simulink model "Rozmyty"  (R2017b)
settings: Solver=ode1  StartTime=0.0  StopTime=3  FixedStep=0.0001  RelTol=1e-3
values from neighbouring files (symbols this model uses):
  Te = 0.001    [Dane_rozmyte.m]
  Tm = 0.2    [Dane_rozmyte.m]
libraries: fuzblock x48
settings Model: Creator=kamil  LastModifiedBy=kamil

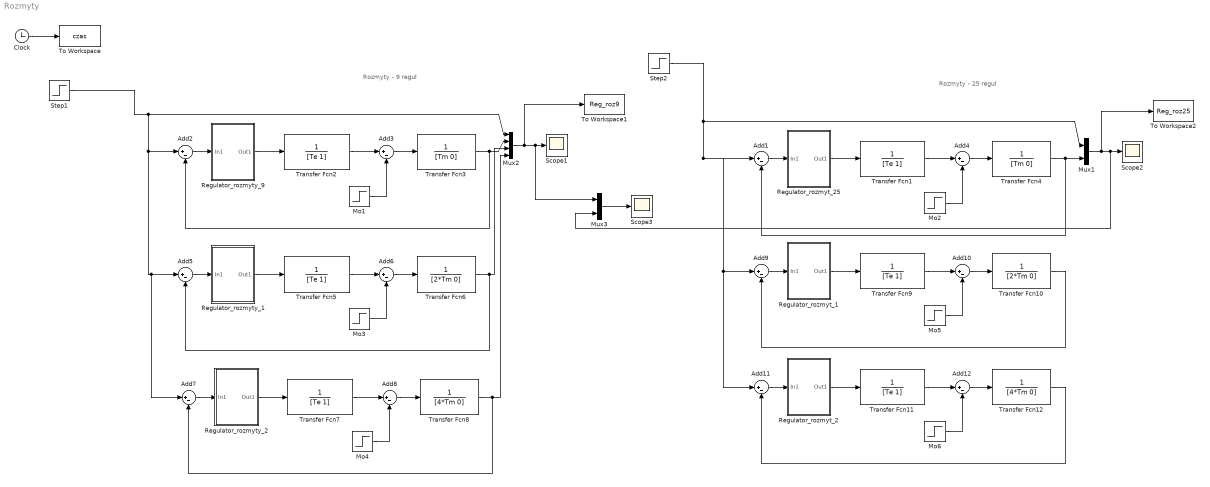
== system Rozmyty ==
  note: Rozmyty - 9 reguł
  note: Rozmyty - 25 reguł
  Add{1..12} (12 alike) : Sum  Inputs=|+-
  Clock : Clock
  Mo{1..6} (6 alike) : Step  Time=2  After=0.5  SampleTime=0
  Mux1 : Mux  Inputs=2
  Mux2 : Mux
  Mux3 : Mux  Inputs=2
  Regulator_rozmyt_1 : Subsystem
  Regulator_rozmyt_2 : Subsystem
  Regulator_rozmyt_25 : Subsystem
  Regulator_rozmyty_1 : Subsystem
  Regulator_rozmyty_2 : Subsystem
  Regulator_rozmyty_9 : Subsystem
  Scope1 : Scope
  Scope2 : Scope
  Scope3 : Scope
  Step1 : Step  After=0.25  SampleTime=0
  Step2 : Step  After=0.25  SampleTime=0
  To Workspace : ToWorkspace  VariableName=czas  SampleTime=-1
  To Workspace1 : ToWorkspace  VariableName=Reg_roz9  SampleTime=-1
  To Workspace2 : ToWorkspace  VariableName=Reg_roz25  SampleTime=-1
  Transfer Fcn{1..2,5,7,9,11} (6 alike) : TransferFcn  Denominator=[Te 1]
  Transfer Fcn10 : TransferFcn  Denominator=[2*Tm 0]
  Transfer Fcn12 : TransferFcn  Denominator=[4*Tm 0]
  Transfer Fcn3 : TransferFcn  Denominator=[Tm 0]
  Transfer Fcn4 : TransferFcn  Denominator=[Tm 0]
  Transfer Fcn6 : TransferFcn  Denominator=[2*Tm 0]
  Transfer Fcn8 : TransferFcn  Denominator=[4*Tm 0]
  wires:
  Add2/1 -> Regulator_rozmyty_9/1(In1)
  Add3/1 -> Transfer Fcn3/1
  Mux2/1 -> To Workspace1/1, Mux3/1, Scope1/1
  Transfer Fcn3/1 -> Mux2/2, Add2/2
  Mo1/1 -> Add3/2
  Transfer Fcn2/1 -> Add3/1
  Regulator_rozmyty_9/1(Out1) -> Transfer Fcn2/1
  Clock/1 -> To Workspace/1
  Regulator_rozmyt_25/1(Out1) -> Transfer Fcn1/1
  Add1/1 -> Regulator_rozmyt_25/1(In1)
  Transfer Fcn1/1 -> Add4/1
  Mo2/1 -> Add4/2
  Add4/1 -> Transfer Fcn4/1
  Mux1/1 -> To Workspace2/1, Mux3/2, Scope2/1
  Transfer Fcn4/1 -> Mux1/2, Add1/2
  Transfer Fcn6/1 -> Mux2/3, Add5/2
  Add5/1 -> Regulator_rozmyty_1/1(In1)
  Mo3/1 -> Add6/2
  Regulator_rozmyty_1/1(Out1) -> Transfer Fcn5/1
  Add6/1 -> Transfer Fcn6/1
  Transfer Fcn5/1 -> Add6/1
  Transfer Fcn8/1 -> Mux2/4, Add7/2
  Step1/1 -> Mux2/1, Add7/1, Add5/1, Add2/1
  Add7/1 -> Regulator_rozmyty_2/1(In1)
  Mo4/1 -> Add8/2
  Regulator_rozmyty_2/1(Out1) -> Transfer Fcn7/1
  Add8/1 -> Transfer Fcn8/1
  Transfer Fcn7/1 -> Add8/1
  Transfer Fcn10/1 -> Add9/2
  Regulator_rozmyt_1/1(Out1) -> Transfer Fcn9/1
  Add10/1 -> Transfer Fcn10/1
  Mo5/1 -> Add10/2
  Transfer Fcn9/1 -> Add10/1
  Add9/1 -> Regulator_rozmyt_1/1(In1)
  Step2/1 -> Mux1/1, Add11/1, Add9/1, Add1/1
  Transfer Fcn12/1 -> Add11/2
  Regulator_rozmyt_2/1(Out1) -> Transfer Fcn11/1
  Add12/1 -> Transfer Fcn12/1
  Mo6/1 -> Add12/2
  Transfer Fcn11/1 -> Add12/1
  Add11/1 -> Regulator_rozmyt_2/1(In1)
  Mux3/1 -> Scope3/1

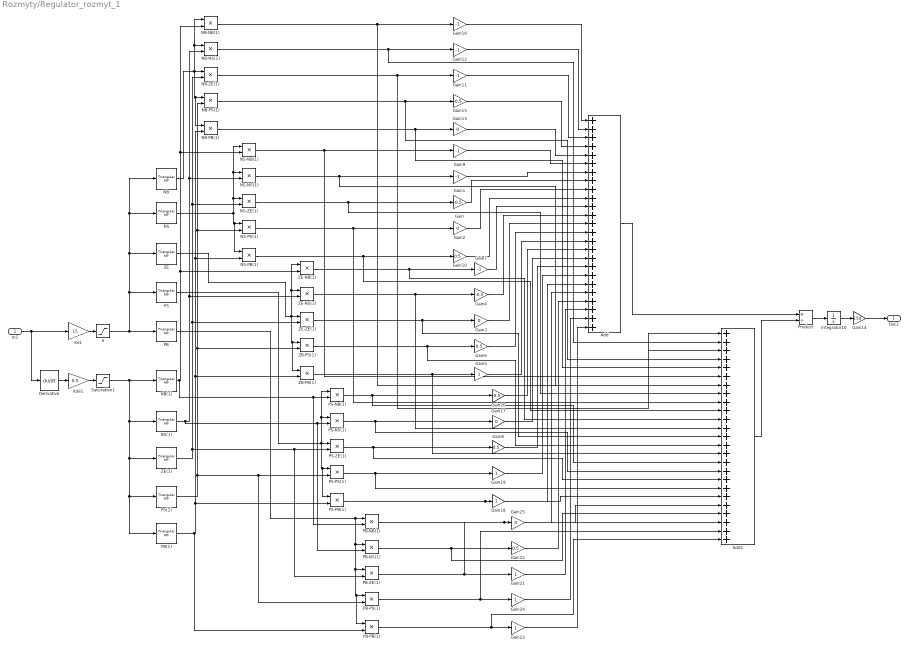
== system Rozmyty/Regulator_rozmyt_1 ==
  In1 : Inport
  Add : Sum  Inputs=+++++++++++++++++++++++++
  Add1 : Sum  Inputs=+++++++++++++++++++++++++
  Derivative : Derivative
  Gain{,4,15,20} (4 alike) : Gain  Gain=-0.5
  Gain{1,7,9,11..12,16} (6 alike) : Gain  Gain=-1
  Gain{6,8,10,22} (4 alike) : Gain  Gain=0.5
  Gain{2..3,13,17,25} (5 alike) : Gain  Gain=0
  Gain14 : Gain  Gain=150
  Gain{5,18..19,21,23..24} (6 alike) : Gain
  Integrator10 : Integrator
  Kde1 : Gain  Gain=0.5
  Ke1 : Gain  Gain=15
  NB : fuzblock/Membership  Functions/Triangular MF  a=-1.5  b=-1  c=-0.5
      settings: SourceProductName=Fuzzy Logic Toolbox  SourceProductBaseCode=FL
  NB(1) : fuzblock/Membership  Functions/Triangular MF  a=-1.5  b=-1  c=-0.5
      settings: SourceProductName=Fuzzy Logic Toolbox  SourceProductBaseCode=FL
  NB-NB(1) : Product
  NB-NS(1) : Product
  NB-PB(1) : Product
  NB-PS(1) : Product
  NB-ZE(1) : Product
  NS : fuzblock/Membership  Functions/Triangular MF  a=-1  b=-0.5  c=0
      settings: SourceProductName=Fuzzy Logic Toolbox  SourceProductBaseCode=FL
  NS(1) : fuzblock/Membership  Functions/Triangular MF  a=-1  b=-0.5  c=0
      settings: SourceProductName=Fuzzy Logic Toolbox  SourceProductBaseCode=FL
  NS-NB(1) : Product
  NS-NS(1) : Product
  NS-PB(1) : Product
  NS-PS(1) : Product
  NS-ZE(1) : Product
  PB : fuzblock/Membership  Functions/Triangular MF  a=0.5  b=1  c=1.5
      settings: SourceProductName=Fuzzy Logic Toolbox  SourceProductBaseCode=FL
  PB(1) : fuzblock/Membership  Functions/Triangular MF  a=0.5  b=1  c=1.5
      settings: SourceProductName=Fuzzy Logic Toolbox  SourceProductBaseCode=FL
  PB-NB(1) : Product
  PB-NS(1) : Product
  PB-PB(1) : Product
  PB-PS(1) : Product
  PB-ZE(1) : Product
  PS : fuzblock/Membership  Functions/Triangular MF  a=0  b=0.5  c=1
      settings: SourceProductName=Fuzzy Logic Toolbox  SourceProductBaseCode=FL
  PS(1) : fuzblock/Membership  Functions/Triangular MF  a=0  b=0.5  c=1
      settings: SourceProductName=Fuzzy Logic Toolbox  SourceProductBaseCode=FL
  PS-NB(1) : Product
  PS-NS(1) : Product
  PS-PB(1) : Product
  PS-PS(1) : Product
  PS-ZE(1) : Product
  Product : Product  Inputs=*/
  Saturation1 : Saturate  UpperLimit=1  LowerLimit=-1
  ZB-PB(1) : Product
  ZB-PS(1) : Product
  ZE : fuzblock/Membership  Functions/Triangular MF  a=-0.5  b=0  c=0.5
      settings: SourceProductName=Fuzzy Logic Toolbox  SourceProductBaseCode=FL
  ZE(1) : fuzblock/Membership  Functions/Triangular MF  a=-0.5  b=0  c=0.5
      settings: SourceProductName=Fuzzy Logic Toolbox  SourceProductBaseCode=FL
  ZE-NB(1) : Product
  ZE-NS(1) : Product
  ZE-ZE(1) : Product
  e : Saturate  UpperLimit=1  LowerLimit=-1
  Out1 : Outport
  wires:
  Ke1/1 -> e/1
  Kde1/1 -> Saturation1/1
  Derivative/1 -> Kde1/1
  In1/1 -> Derivative/1, Ke1/1
  e/1 -> PB/1, PS/1, NB/1, NS/1, ZE/1
  Saturation1/1 -> NB(1)/1, NS(1)/1, PB(1)/1, PS(1)/1, ZE(1)/1
  NS/1 -> NS-NB(1)/1, NS-NS(1)/1, NS-ZE(1)/1, NS-PB(1)/1, NS-PS(1)/1
  NS-NS(1)/1 -> Add1/7, Gain1/1
  NS-ZE(1)/1 -> Add1/8, Gain/1
  NS-PS(1)/1 -> Add1/9, Gain2/1
  Add/1 -> Product/1
  Add1/1 -> Product/2
  Integrator10/1 -> Gain14/1
  Product/1 -> Integrator10/1
  Gain14/1 -> Out1/1
  NS-NB(1)/1 -> Add1/6, Gain9/1
  NS-PB(1)/1 -> Add1/10, Gain10/1
  NB-PS(1)/1 -> Add1/4, Gain15/1
  NB/1 -> NB-NB(1)/1, NB-NS(1)/1, NB-ZE(1)/1, NB-PB(1)/1, NB-PS(1)/1
  NB-ZE(1)/1 -> Add1/3, Gain11/1
  NB-NB(1)/1 -> Add1/1, Gain16/1
  NB-NS(1)/1 -> Add1/2, Gain12/1
  NB-PB(1)/1 -> Add1/5, Gain13/1
  ZE-NS(1)/1 -> Add1/12, Gain4/1
  ZE-ZE(1)/1 -> Add1/13, Gain3/1
  ZB-PB(1)/1 -> Add1/15, Gain5/1
  ZE/1 -> ZE-NB(1)/1, ZE-NS(1)/1, ZE-ZE(1)/1, ZB-PB(1)/1, ZB-PS(1)/1
  ZE-NB(1)/1 -> Add1/11, Gain7/1
  ZB-PS(1)/1 -> Add1/14, Gain6/1
  PS-NS(1)/1 -> Add1/17, Gain17/1
  PS-ZE(1)/1 -> Add1/18, Gain8/1
  PS-PB(1)/1 -> Add1/20, Gain18/1
  PS/1 -> PS-NB(1)/1, PS-NS(1)/1, PS-ZE(1)/1, PS-PB(1)/1, PS-PS(1)/1
  PS-NB(1)/1 -> Add1/16, Gain20/1
  PB-NS(1)/1 -> Add1/22, Gain22/1
  PB-ZE(1)/1 -> Add1/23, Gain21/1
  PB-PB(1)/1 -> Add1/25, Gain23/1
  PB/1 -> PB-ZE(1)/1, PB-PB(1)/1, PB-PS(1)/1, PB-NS(1)/1, PB-NB(1)/1
  PB-NB(1)/1 -> Add1/21, Gain25/1
  PB-PS(1)/1 -> Add1/24, Gain24/1
  NB(1)/1 -> PB-NB(1)/2, PS-NB(1)/2, ZE-NB(1)/2, NS-NB(1)/2, NB-NB(1)/2
  NS(1)/1 -> PB-NS(1)/2, PS-NS(1)/2, ZE-NS(1)/2, NS-NS(1)/2, NB-NS(1)/2
  ZE(1)/1 -> PB-ZE(1)/2, PS-ZE(1)/2, ZE-ZE(1)/2, NS-ZE(1)/2, NB-ZE(1)/2
  PS(1)/1 -> PB-PS(1)/2, PS-PS(1)/2, ZB-PS(1)/2, NS-PS(1)/2, NB-PS(1)/2
  PB(1)/1 -> PB-PB(1)/2, PS-PB(1)/2, ZB-PB(1)/2, NS-PB(1)/2, NB-PB(1)/2
  Gain16/1 -> Add/1
  Gain12/1 -> Add/2
  Gain11/1 -> Add/3
  Gain15/1 -> Add/4
  Gain13/1 -> Add/5
  Gain9/1 -> Add/6
  Gain1/1 -> Add/7
  Gain/1 -> Add/8
  Gain2/1 -> Add/9
  Gain10/1 -> Add/10
  Gain7/1 -> Add/11
  Gain4/1 -> Add/12
  Gain3/1 -> Add/13
  Gain6/1 -> Add/14
  Gain5/1 -> Add/15
  Gain20/1 -> Add/16
  Gain17/1 -> Add/17
  Gain8/1 -> Add/18
  Gain19/1 -> Add/19
  Gain18/1 -> Add/20
  Gain25/1 -> Add/21
  Gain22/1 -> Add/22
  Gain21/1 -> Add/23
  Gain23/1 -> Add/25
  Gain24/1 -> Add/24
  PS-PS(1)/1 -> Add1/19, Gain19/1

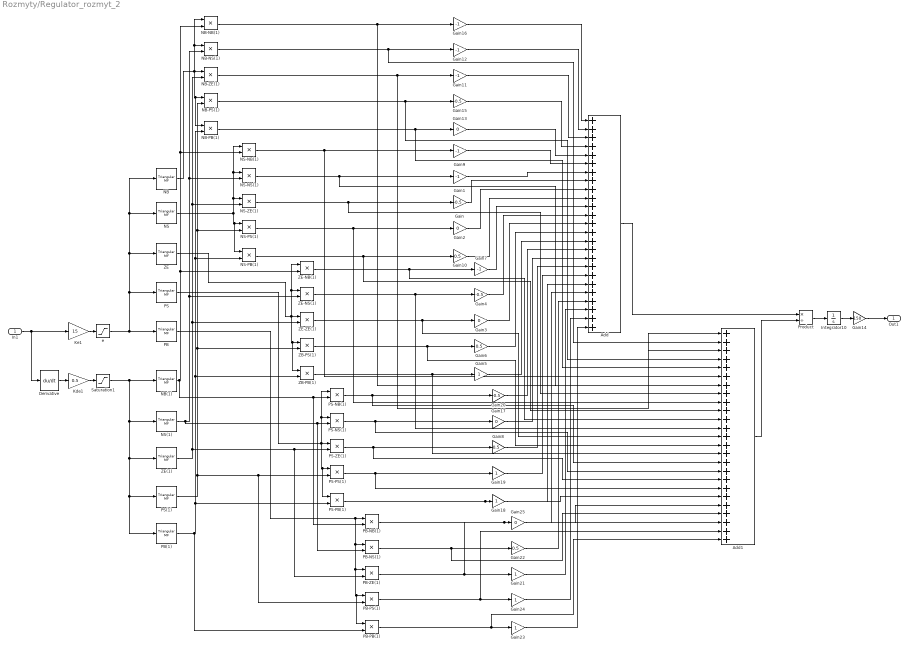
== system Rozmyty/Regulator_rozmyt_2 ==
  In1 : Inport
  Add : Sum  Inputs=+++++++++++++++++++++++++
  Add1 : Sum  Inputs=+++++++++++++++++++++++++
  Derivative : Derivative
  Gain{,4,15,20} (4 alike) : Gain  Gain=-0.5
  Gain{1,7,9,11..12,16} (6 alike) : Gain  Gain=-1
  Gain{6,8,10,22} (4 alike) : Gain  Gain=0.5
  Gain{2..3,13,17,25} (5 alike) : Gain  Gain=0
  Gain14 : Gain  Gain=150
  Gain{5,18..19,21,23..24} (6 alike) : Gain
  Integrator10 : Integrator
  Kde1 : Gain  Gain=0.5
  Ke1 : Gain  Gain=15
  NB : fuzblock/Membership  Functions/Triangular MF  a=-1.5  b=-1  c=-0.5
      settings: SourceProductName=Fuzzy Logic Toolbox  SourceProductBaseCode=FL
  NB(1) : fuzblock/Membership  Functions/Triangular MF  a=-1.5  b=-1  c=-0.5
      settings: SourceProductName=Fuzzy Logic Toolbox  SourceProductBaseCode=FL
  NB-NB(1) : Product
  NB-NS(1) : Product
  NB-PB(1) : Product
  NB-PS(1) : Product
  NB-ZE(1) : Product
  NS : fuzblock/Membership  Functions/Triangular MF  a=-1  b=-0.5  c=0
      settings: SourceProductName=Fuzzy Logic Toolbox  SourceProductBaseCode=FL
  NS(1) : fuzblock/Membership  Functions/Triangular MF  a=-1  b=-0.5  c=0
      settings: SourceProductName=Fuzzy Logic Toolbox  SourceProductBaseCode=FL
  NS-NB(1) : Product
  NS-NS(1) : Product
  NS-PB(1) : Product
  NS-PS(1) : Product
  NS-ZE(1) : Product
  PB : fuzblock/Membership  Functions/Triangular MF  a=0.5  b=1  c=1.5
      settings: SourceProductName=Fuzzy Logic Toolbox  SourceProductBaseCode=FL
  PB(1) : fuzblock/Membership  Functions/Triangular MF  a=0.5  b=1  c=1.5
      settings: SourceProductName=Fuzzy Logic Toolbox  SourceProductBaseCode=FL
  PB-NB(1) : Product
  PB-NS(1) : Product
  PB-PB(1) : Product
  PB-PS(1) : Product
  PB-ZE(1) : Product
  PS : fuzblock/Membership  Functions/Triangular MF  a=0  b=0.5  c=1
      settings: SourceProductName=Fuzzy Logic Toolbox  SourceProductBaseCode=FL
  PS(1) : fuzblock/Membership  Functions/Triangular MF  a=0  b=0.5  c=1
      settings: SourceProductName=Fuzzy Logic Toolbox  SourceProductBaseCode=FL
  PS-NB(1) : Product
  PS-NS(1) : Product
  PS-PB(1) : Product
  PS-PS(1) : Product
  PS-ZE(1) : Product
  Product : Product  Inputs=*/
  Saturation1 : Saturate  UpperLimit=1  LowerLimit=-1
  ZB-PB(1) : Product
  ZB-PS(1) : Product
  ZE : fuzblock/Membership  Functions/Triangular MF  a=-0.5  b=0  c=0.5
      settings: SourceProductName=Fuzzy Logic Toolbox  SourceProductBaseCode=FL
  ZE(1) : fuzblock/Membership  Functions/Triangular MF  a=-0.5  b=0  c=0.5
      settings: SourceProductName=Fuzzy Logic Toolbox  SourceProductBaseCode=FL
  ZE-NB(1) : Product
  ZE-NS(1) : Product
  ZE-ZE(1) : Product
  e : Saturate  UpperLimit=1  LowerLimit=-1
  Out1 : Outport
  wires:
  Ke1/1 -> e/1
  Kde1/1 -> Saturation1/1
  Derivative/1 -> Kde1/1
  In1/1 -> Derivative/1, Ke1/1
  e/1 -> PB/1, PS/1, NB/1, NS/1, ZE/1
  Saturation1/1 -> NB(1)/1, NS(1)/1, PB(1)/1, PS(1)/1, ZE(1)/1
  NS/1 -> NS-NB(1)/1, NS-NS(1)/1, NS-ZE(1)/1, NS-PB(1)/1, NS-PS(1)/1
  NS-NS(1)/1 -> Add1/7, Gain1/1
  NS-ZE(1)/1 -> Add1/8, Gain/1
  NS-PS(1)/1 -> Add1/9, Gain2/1
  Add/1 -> Product/1
  Add1/1 -> Product/2
  Integrator10/1 -> Gain14/1
  Product/1 -> Integrator10/1
  Gain14/1 -> Out1/1
  NS-NB(1)/1 -> Add1/6, Gain9/1
  NS-PB(1)/1 -> Add1/10, Gain10/1
  NB-PS(1)/1 -> Add1/4, Gain15/1
  NB/1 -> NB-NB(1)/1, NB-NS(1)/1, NB-ZE(1)/1, NB-PB(1)/1, NB-PS(1)/1
  NB-ZE(1)/1 -> Add1/3, Gain11/1
  NB-NB(1)/1 -> Add1/1, Gain16/1
  NB-NS(1)/1 -> Add1/2, Gain12/1
  NB-PB(1)/1 -> Add1/5, Gain13/1
  ZE-NS(1)/1 -> Add1/12, Gain4/1
  ZE-ZE(1)/1 -> Add1/13, Gain3/1
  ZB-PB(1)/1 -> Add1/15, Gain5/1
  ZE/1 -> ZE-NB(1)/1, ZE-NS(1)/1, ZE-ZE(1)/1, ZB-PB(1)/1, ZB-PS(1)/1
  ZE-NB(1)/1 -> Add1/11, Gain7/1
  ZB-PS(1)/1 -> Add1/14, Gain6/1
  PS-NS(1)/1 -> Add1/17, Gain17/1
  PS-ZE(1)/1 -> Add1/18, Gain8/1
  PS-PB(1)/1 -> Add1/20, Gain18/1
  PS/1 -> PS-NB(1)/1, PS-NS(1)/1, PS-ZE(1)/1, PS-PB(1)/1, PS-PS(1)/1
  PS-NB(1)/1 -> Add1/16, Gain20/1
  PB-NS(1)/1 -> Add1/22, Gain22/1
  PB-ZE(1)/1 -> Add1/23, Gain21/1
  PB-PB(1)/1 -> Add1/25, Gain23/1
  PB/1 -> PB-ZE(1)/1, PB-PB(1)/1, PB-PS(1)/1, PB-NS(1)/1, PB-NB(1)/1
  PB-NB(1)/1 -> Add1/21, Gain25/1
  PB-PS(1)/1 -> Add1/24, Gain24/1
  NB(1)/1 -> PB-NB(1)/2, PS-NB(1)/2, ZE-NB(1)/2, NS-NB(1)/2, NB-NB(1)/2
  NS(1)/1 -> PB-NS(1)/2, PS-NS(1)/2, ZE-NS(1)/2, NS-NS(1)/2, NB-NS(1)/2
  ZE(1)/1 -> PB-ZE(1)/2, PS-ZE(1)/2, ZE-ZE(1)/2, NS-ZE(1)/2, NB-ZE(1)/2
  PS(1)/1 -> PB-PS(1)/2, PS-PS(1)/2, ZB-PS(1)/2, NS-PS(1)/2, NB-PS(1)/2
  PB(1)/1 -> PB-PB(1)/2, PS-PB(1)/2, ZB-PB(1)/2, NS-PB(1)/2, NB-PB(1)/2
  Gain16/1 -> Add/1
  Gain12/1 -> Add/2
  Gain11/1 -> Add/3
  Gain15/1 -> Add/4
  Gain13/1 -> Add/5
  Gain9/1 -> Add/6
  Gain1/1 -> Add/7
  Gain/1 -> Add/8
  Gain2/1 -> Add/9
  Gain10/1 -> Add/10
  Gain7/1 -> Add/11
  Gain4/1 -> Add/12
  Gain3/1 -> Add/13
  Gain6/1 -> Add/14
  Gain5/1 -> Add/15
  Gain20/1 -> Add/16
  Gain17/1 -> Add/17
  Gain8/1 -> Add/18
  Gain19/1 -> Add/19
  Gain18/1 -> Add/20
  Gain25/1 -> Add/21
  Gain22/1 -> Add/22
  Gain21/1 -> Add/23
  Gain23/1 -> Add/25
  Gain24/1 -> Add/24
  PS-PS(1)/1 -> Add1/19, Gain19/1

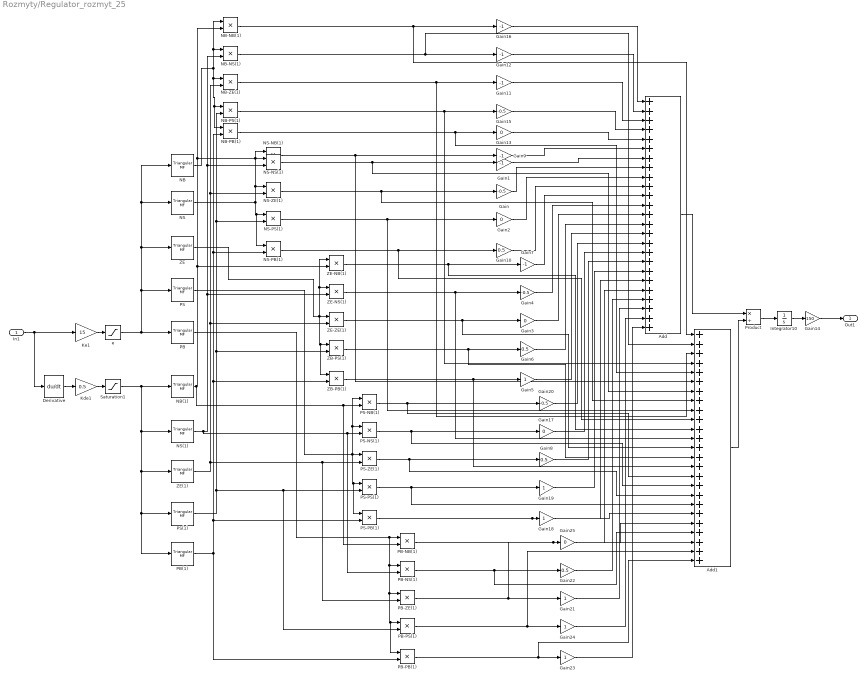
== system Rozmyty/Regulator_rozmyt_25 ==
  In1 : Inport
  Add : Sum  Inputs=+++++++++++++++++++++++++
  Add1 : Sum  Inputs=+++++++++++++++++++++++++
  Derivative : Derivative
  Gain{,4,15,20} (4 alike) : Gain  Gain=-0.5
  Gain{1,7,9,11..12,16} (6 alike) : Gain  Gain=-1
  Gain{6,8,10,22} (4 alike) : Gain  Gain=0.5
  Gain{2..3,13,17,25} (5 alike) : Gain  Gain=0
  Gain14 : Gain  Gain=150
  Gain{5,18..19,21,23..24} (6 alike) : Gain
  Integrator10 : Integrator
  Kde1 : Gain  Gain=0.5
  Ke1 : Gain  Gain=15
  NB : fuzblock/Membership  Functions/Triangular MF  a=-1.5  b=-1  c=-0.5
      settings: SourceProductName=Fuzzy Logic Toolbox  SourceProductBaseCode=FL
  NB(1) : fuzblock/Membership  Functions/Triangular MF  a=-1.5  b=-1  c=-0.5
      settings: SourceProductName=Fuzzy Logic Toolbox  SourceProductBaseCode=FL
  NB-NB(1) : Product
  NB-NS(1) : Product
  NB-PB(1) : Product
  NB-PS(1) : Product
  NB-ZE(1) : Product
  NS : fuzblock/Membership  Functions/Triangular MF  a=-1  b=-0.5  c=0
      settings: SourceProductName=Fuzzy Logic Toolbox  SourceProductBaseCode=FL
  NS(1) : fuzblock/Membership  Functions/Triangular MF  a=-1  b=-0.5  c=0
      settings: SourceProductName=Fuzzy Logic Toolbox  SourceProductBaseCode=FL
  NS-NB(1) : Product
  NS-NS(1) : Product
  NS-PB(1) : Product
  NS-PS(1) : Product
  NS-ZE(1) : Product
  PB : fuzblock/Membership  Functions/Triangular MF  a=0.5  b=1  c=1.5
      settings: SourceProductName=Fuzzy Logic Toolbox  SourceProductBaseCode=FL
  PB(1) : fuzblock/Membership  Functions/Triangular MF  a=0.5  b=1  c=1.5
      settings: SourceProductName=Fuzzy Logic Toolbox  SourceProductBaseCode=FL
  PB-NB(1) : Product
  PB-NS(1) : Product
  PB-PB(1) : Product
  PB-PS(1) : Product
  PB-ZE(1) : Product
  PS : fuzblock/Membership  Functions/Triangular MF  a=0  b=0.5  c=1
      settings: SourceProductName=Fuzzy Logic Toolbox  SourceProductBaseCode=FL
  PS(1) : fuzblock/Membership  Functions/Triangular MF  a=0  b=0.5  c=1
      settings: SourceProductName=Fuzzy Logic Toolbox  SourceProductBaseCode=FL
  PS-NB(1) : Product
  PS-NS(1) : Product
  PS-PB(1) : Product
  PS-PS(1) : Product
  PS-ZE(1) : Product
  Product : Product  Inputs=*/
  Saturation1 : Saturate  UpperLimit=1  LowerLimit=-1
  ZB-PB(1) : Product
  ZB-PS(1) : Product
  ZE : fuzblock/Membership  Functions/Triangular MF  a=-0.5  b=0  c=0.5
      settings: SourceProductName=Fuzzy Logic Toolbox  SourceProductBaseCode=FL
  ZE(1) : fuzblock/Membership  Functions/Triangular MF  a=-0.5  b=0  c=0.5
      settings: SourceProductName=Fuzzy Logic Toolbox  SourceProductBaseCode=FL
  ZE-NB(1) : Product
  ZE-NS(1) : Product
  ZE-ZE(1) : Product
  e : Saturate  UpperLimit=1  LowerLimit=-1
  Out1 : Outport
  wires:
  Ke1/1 -> e/1
  Kde1/1 -> Saturation1/1
  Derivative/1 -> Kde1/1
  In1/1 -> Derivative/1, Ke1/1
  e/1 -> PB/1, PS/1, NB/1, NS/1, ZE/1
  Saturation1/1 -> NB(1)/1, NS(1)/1, PB(1)/1, PS(1)/1, ZE(1)/1
  NS/1 -> NS-NB(1)/1, NS-NS(1)/1, NS-ZE(1)/1, NS-PB(1)/1, NS-PS(1)/1
  NS-NS(1)/1 -> Add1/7, Gain1/1
  NS-ZE(1)/1 -> Add1/8, Gain/1
  NS-PS(1)/1 -> Add1/9, Gain2/1
  Add/1 -> Product/1
  Add1/1 -> Product/2
  Integrator10/1 -> Gain14/1
  Product/1 -> Integrator10/1
  Gain14/1 -> Out1/1
  NS-NB(1)/1 -> Add1/6, Gain9/1
  NS-PB(1)/1 -> Add1/10, Gain10/1
  NB-PS(1)/1 -> Add1/4, Gain15/1
  NB/1 -> NB-ZE(1)/1, NB-PB(1)/1, NB-PS(1)/1, NB-NB(1)/1, NB-NS(1)/1
  NB-ZE(1)/1 -> Add1/3, Gain11/1
  NB-NB(1)/1 -> Add1/1, Gain16/1
  NB-NS(1)/1 -> Add1/2, Gain12/1
  NB-PB(1)/1 -> Add1/5, Gain13/1
  ZE-NS(1)/1 -> Add1/12, Gain4/1
  ZE-ZE(1)/1 -> Add1/13, Gain3/1
  ZB-PB(1)/1 -> Add1/15, Gain5/1
  ZE/1 -> ZE-NB(1)/1, ZE-NS(1)/1, ZE-ZE(1)/1, ZB-PB(1)/1, ZB-PS(1)/1
  ZE-NB(1)/1 -> Add1/11, Gain7/1
  ZB-PS(1)/1 -> Add1/14, Gain6/1
  PS-NS(1)/1 -> Add1/17, Gain17/1
  PS-ZE(1)/1 -> Add1/18, Gain8/1
  PS-PB(1)/1 -> Add1/20, Gain18/1
  PS/1 -> PS-NB(1)/1, PS-NS(1)/1, PS-ZE(1)/1, PS-PB(1)/1, PS-PS(1)/1
  PS-NB(1)/1 -> Add1/16, Gain20/1
  PB-NS(1)/1 -> Add1/22, Gain22/1
  PB-ZE(1)/1 -> Add1/23, Gain21/1
  PB-PB(1)/1 -> Add1/25, Gain23/1
  PB/1 -> PB-ZE(1)/1, PB-PB(1)/1, PB-PS(1)/1, PB-NS(1)/1, PB-NB(1)/1
  PB-NB(1)/1 -> Add1/21, Gain25/1
  PB-PS(1)/1 -> Add1/24, Gain24/1
  NB(1)/1 -> PB-NB(1)/2, PS-NB(1)/2, ZE-NB(1)/2, NS-NB(1)/2, NB-NB(1)/2
  NS(1)/1 -> PB-NS(1)/2, PS-NS(1)/2, ZE-NS(1)/2, NS-NS(1)/2, NB-NS(1)/2
  ZE(1)/1 -> PB-ZE(1)/2, PS-ZE(1)/2, ZE-ZE(1)/2, NS-ZE(1)/2, NB-ZE(1)/2
  PS(1)/1 -> PB-PS(1)/2, PS-PS(1)/2, ZB-PS(1)/2, NS-PS(1)/2, NB-PS(1)/2
  PB(1)/1 -> PB-PB(1)/2, PS-PB(1)/2, ZB-PB(1)/2, NS-PB(1)/2, NB-PB(1)/2
  Gain16/1 -> Add/1
  Gain12/1 -> Add/2
  Gain11/1 -> Add/3
  Gain15/1 -> Add/4
  Gain13/1 -> Add/5
  Gain9/1 -> Add/6
  Gain1/1 -> Add/7
  Gain/1 -> Add/8
  Gain2/1 -> Add/9
  Gain10/1 -> Add/10
  Gain7/1 -> Add/11
  Gain4/1 -> Add/12
  Gain3/1 -> Add/13
  Gain6/1 -> Add/14
  Gain5/1 -> Add/15
  Gain20/1 -> Add/16
  Gain17/1 -> Add/17
  Gain8/1 -> Add/18
  Gain19/1 -> Add/19
  Gain18/1 -> Add/20
  Gain25/1 -> Add/21
  Gain22/1 -> Add/22
  Gain21/1 -> Add/23
  Gain23/1 -> Add/25
  Gain24/1 -> Add/24
  PS-PS(1)/1 -> Add1/19, Gain19/1

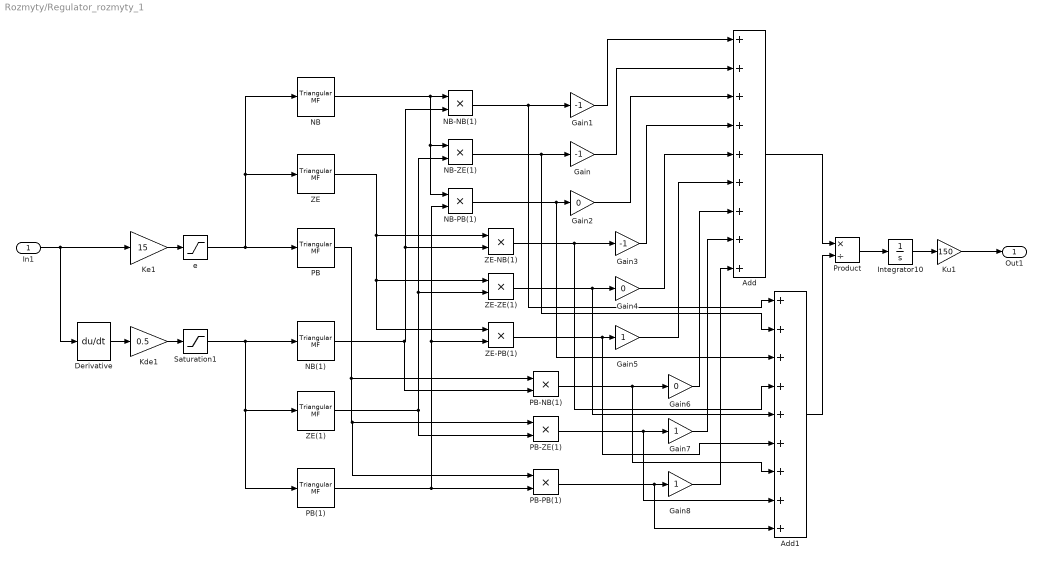
== system Rozmyty/Regulator_rozmyty_1 ==
  In1 : Inport
  Add : Sum  Inputs=+++++++++
  Add1 : Sum  Inputs=+++++++++
  Derivative : Derivative
  Gain : Gain  Gain=-1
  Gain1 : Gain  Gain=-1
  Gain2 : Gain  Gain=0
  Gain3 : Gain  Gain=-1
  Gain4 : Gain  Gain=0
  Gain5 : Gain
  Gain6 : Gain  Gain=0
  Gain7 : Gain
  Gain8 : Gain
  Integrator10 : Integrator
  Kde1 : Gain  Gain=0.5
  Ke1 : Gain  Gain=15
  Ku1 : Gain  Gain=150
  NB : fuzblock/Membership  Functions/Triangular MF  a=-2  b=-1  c=0
      settings: SourceProductName=Fuzzy Logic Toolbox  SourceProductBaseCode=FL
  NB(1) : fuzblock/Membership  Functions/Triangular MF  a=-2  b=-1  c=0
      settings: SourceProductName=Fuzzy Logic Toolbox  SourceProductBaseCode=FL
  NB-NB(1) : Product
  NB-PB(1) : Product
  NB-ZE(1) : Product
  PB : fuzblock/Membership  Functions/Triangular MF  a=0  b=1  c=2
      settings: SourceProductName=Fuzzy Logic Toolbox  SourceProductBaseCode=FL
  PB(1) : fuzblock/Membership  Functions/Triangular MF  a=0  b=1  c=2
      settings: SourceProductName=Fuzzy Logic Toolbox  SourceProductBaseCode=FL
  PB-NB(1) : Product
  PB-PB(1) : Product
  PB-ZE(1) : Product
  Product : Product  Inputs=*/
  Saturation1 : Saturate  UpperLimit=1  LowerLimit=-1
  ZE : fuzblock/Membership  Functions/Triangular MF  a=-1  b=0  c=1
      settings: SourceProductName=Fuzzy Logic Toolbox  SourceProductBaseCode=FL
  ZE(1) : fuzblock/Membership  Functions/Triangular MF  a=-1  b=0  c=1
      settings: SourceProductName=Fuzzy Logic Toolbox  SourceProductBaseCode=FL
  ZE-NB(1) : Product
  ZE-PB(1) : Product
  ZE-ZE(1) : Product
  e : Saturate  UpperLimit=1  LowerLimit=-1
  Out1 : Outport
  wires:
  Ke1/1 -> e/1
  Kde1/1 -> Saturation1/1
  Derivative/1 -> Kde1/1
  In1/1 -> Derivative/1, Ke1/1
  e/1 -> PB/1, NB/1, ZE/1
  Saturation1/1 -> PB(1)/1, ZE(1)/1, NB(1)/1
  NB/1 -> NB-ZE(1)/1, NB-PB(1)/1, NB-NB(1)/1
  NB(1)/1 -> PB-NB(1)/2, NB-NB(1)/2, ZE-NB(1)/2
  ZE(1)/1 -> PB-ZE(1)/2, NB-ZE(1)/2, ZE-ZE(1)/2
  PB(1)/1 -> NB-PB(1)/2, ZE-PB(1)/2, PB-PB(1)/2
  ZE/1 -> ZE-NB(1)/1, ZE-ZE(1)/1, ZE-PB(1)/1
  PB/1 -> PB-NB(1)/1, PB-PB(1)/1, PB-ZE(1)/1
  NB-NB(1)/1 -> Add1/1, Gain1/1
  NB-ZE(1)/1 -> Add1/2, Gain/1
  NB-PB(1)/1 -> Add1/3, Gain2/1
  ZE-NB(1)/1 -> Add1/4, Gain3/1
  ZE-ZE(1)/1 -> Add1/5, Gain4/1
  ZE-PB(1)/1 -> Add1/6, Gain5/1
  PB-NB(1)/1 -> Add1/7, Gain6/1
  PB-ZE(1)/1 -> Add1/8, Gain7/1
  PB-PB(1)/1 -> Add1/9, Gain8/1
  Gain1/1 -> Add/1
  Gain/1 -> Add/2
  Gain2/1 -> Add/3
  Gain3/1 -> Add/4
  Gain4/1 -> Add/5
  Gain5/1 -> Add/6
  Gain6/1 -> Add/7
  Gain7/1 -> Add/8
  Gain8/1 -> Add/9
  Add/1 -> Product/1
  Add1/1 -> Product/2
  Integrator10/1 -> Ku1/1
  Product/1 -> Integrator10/1
  Ku1/1 -> Out1/1

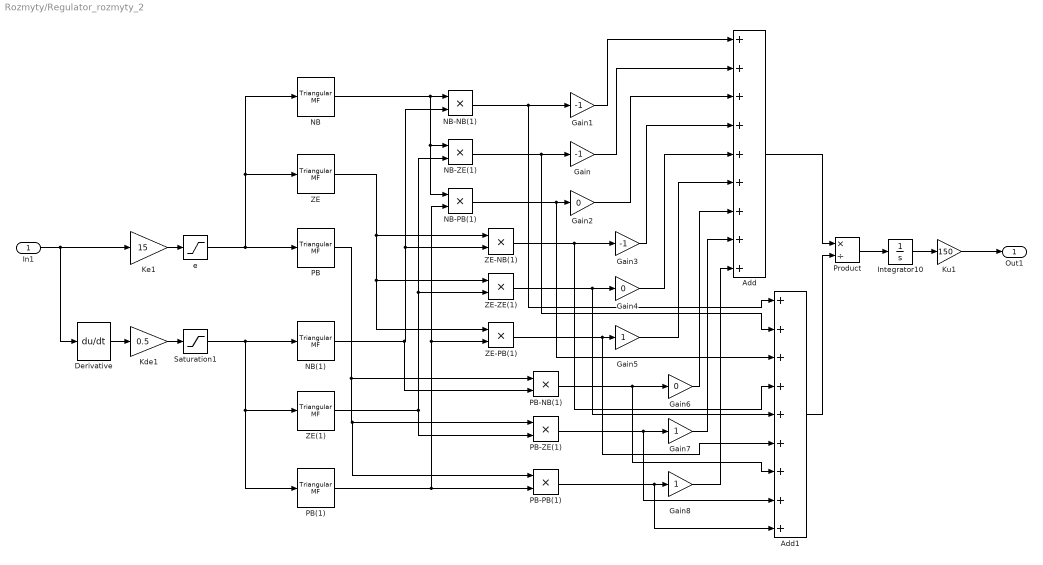
== system Rozmyty/Regulator_rozmyty_2 ==
  In1 : Inport
  Add : Sum  Inputs=+++++++++
  Add1 : Sum  Inputs=+++++++++
  Derivative : Derivative
  Gain : Gain  Gain=-1
  Gain1 : Gain  Gain=-1
  Gain2 : Gain  Gain=0
  Gain3 : Gain  Gain=-1
  Gain4 : Gain  Gain=0
  Gain5 : Gain
  Gain6 : Gain  Gain=0
  Gain7 : Gain
  Gain8 : Gain
  Integrator10 : Integrator
  Kde1 : Gain  Gain=0.5
  Ke1 : Gain  Gain=15
  Ku1 : Gain  Gain=150
  NB : fuzblock/Membership  Functions/Triangular MF  a=-2  b=-1  c=0
      settings: SourceProductName=Fuzzy Logic Toolbox  SourceProductBaseCode=FL
  NB(1) : fuzblock/Membership  Functions/Triangular MF  a=-2  b=-1  c=0
      settings: SourceProductName=Fuzzy Logic Toolbox  SourceProductBaseCode=FL
  NB-NB(1) : Product
  NB-PB(1) : Product
  NB-ZE(1) : Product
  PB : fuzblock/Membership  Functions/Triangular MF  a=0  b=1  c=2
      settings: SourceProductName=Fuzzy Logic Toolbox  SourceProductBaseCode=FL
  PB(1) : fuzblock/Membership  Functions/Triangular MF  a=0  b=1  c=2
      settings: SourceProductName=Fuzzy Logic Toolbox  SourceProductBaseCode=FL
  PB-NB(1) : Product
  PB-PB(1) : Product
  PB-ZE(1) : Product
  Product : Product  Inputs=*/
  Saturation1 : Saturate  UpperLimit=1  LowerLimit=-1
  ZE : fuzblock/Membership  Functions/Triangular MF  a=-1  b=0  c=1
      settings: SourceProductName=Fuzzy Logic Toolbox  SourceProductBaseCode=FL
  ZE(1) : fuzblock/Membership  Functions/Triangular MF  a=-1  b=0  c=1
      settings: SourceProductName=Fuzzy Logic Toolbox  SourceProductBaseCode=FL
  ZE-NB(1) : Product
  ZE-PB(1) : Product
  ZE-ZE(1) : Product
  e : Saturate  UpperLimit=1  LowerLimit=-1
  Out1 : Outport
  wires:
  Ke1/1 -> e/1
  Kde1/1 -> Saturation1/1
  Derivative/1 -> Kde1/1
  In1/1 -> Derivative/1, Ke1/1
  e/1 -> PB/1, NB/1, ZE/1
  Saturation1/1 -> PB(1)/1, ZE(1)/1, NB(1)/1
  NB/1 -> NB-ZE(1)/1, NB-PB(1)/1, NB-NB(1)/1
  NB(1)/1 -> PB-NB(1)/2, NB-NB(1)/2, ZE-NB(1)/2
  ZE(1)/1 -> PB-ZE(1)/2, NB-ZE(1)/2, ZE-ZE(1)/2
  PB(1)/1 -> NB-PB(1)/2, ZE-PB(1)/2, PB-PB(1)/2
  ZE/1 -> ZE-NB(1)/1, ZE-ZE(1)/1, ZE-PB(1)/1
  PB/1 -> PB-NB(1)/1, PB-PB(1)/1, PB-ZE(1)/1
  NB-NB(1)/1 -> Add1/1, Gain1/1
  NB-ZE(1)/1 -> Add1/2, Gain/1
  NB-PB(1)/1 -> Add1/3, Gain2/1
  ZE-NB(1)/1 -> Add1/4, Gain3/1
  ZE-ZE(1)/1 -> Add1/5, Gain4/1
  ZE-PB(1)/1 -> Add1/6, Gain5/1
  PB-NB(1)/1 -> Add1/7, Gain6/1
  PB-ZE(1)/1 -> Add1/8, Gain7/1
  PB-PB(1)/1 -> Add1/9, Gain8/1
  Gain1/1 -> Add/1
  Gain/1 -> Add/2
  Gain2/1 -> Add/3
  Gain3/1 -> Add/4
  Gain4/1 -> Add/5
  Gain5/1 -> Add/6
  Gain6/1 -> Add/7
  Gain7/1 -> Add/8
  Gain8/1 -> Add/9
  Add/1 -> Product/1
  Add1/1 -> Product/2
  Integrator10/1 -> Ku1/1
  Product/1 -> Integrator10/1
  Ku1/1 -> Out1/1

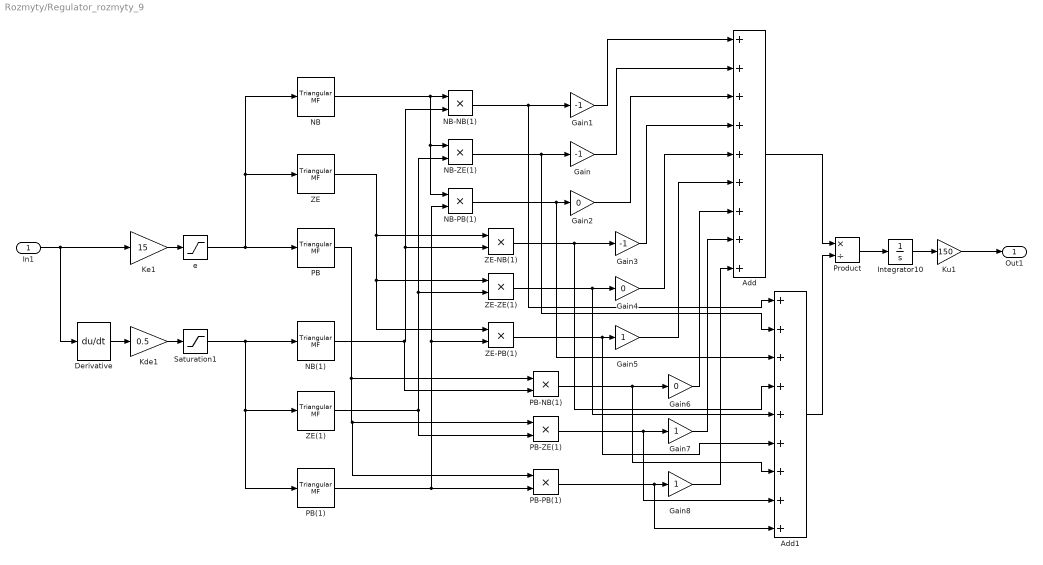
== system Rozmyty/Regulator_rozmyty_9 ==
  In1 : Inport
  Add : Sum  Inputs=+++++++++
  Add1 : Sum  Inputs=+++++++++
  Derivative : Derivative
  Gain : Gain  Gain=-1
  Gain1 : Gain  Gain=-1
  Gain2 : Gain  Gain=0
  Gain3 : Gain  Gain=-1
  Gain4 : Gain  Gain=0
  Gain5 : Gain
  Gain6 : Gain  Gain=0
  Gain7 : Gain
  Gain8 : Gain
  Integrator10 : Integrator
  Kde1 : Gain  Gain=0.5
  Ke1 : Gain  Gain=15
  Ku1 : Gain  Gain=150
  NB : fuzblock/Membership  Functions/Triangular MF  a=-2  b=-1  c=0
      settings: SourceProductName=Fuzzy Logic Toolbox  SourceProductBaseCode=FL
  NB(1) : fuzblock/Membership  Functions/Triangular MF  a=-2  b=-1  c=0
      settings: SourceProductName=Fuzzy Logic Toolbox  SourceProductBaseCode=FL
  NB-NB(1) : Product
  NB-PB(1) : Product
  NB-ZE(1) : Product
  PB : fuzblock/Membership  Functions/Triangular MF  a=0  b=1  c=2
      settings: SourceProductName=Fuzzy Logic Toolbox  SourceProductBaseCode=FL
  PB(1) : fuzblock/Membership  Functions/Triangular MF  a=0  b=1  c=2
      settings: SourceProductName=Fuzzy Logic Toolbox  SourceProductBaseCode=FL
  PB-NB(1) : Product
  PB-PB(1) : Product
  PB-ZE(1) : Product
  Product : Product  Inputs=*/
  Saturation1 : Saturate  UpperLimit=1  LowerLimit=-1
  ZE : fuzblock/Membership  Functions/Triangular MF  a=-1  b=0  c=1
      settings: SourceProductName=Fuzzy Logic Toolbox  SourceProductBaseCode=FL
  ZE(1) : fuzblock/Membership  Functions/Triangular MF  a=-1  b=0  c=1
      settings: SourceProductName=Fuzzy Logic Toolbox  SourceProductBaseCode=FL
  ZE-NB(1) : Product
  ZE-PB(1) : Product
  ZE-ZE(1) : Product
  e : Saturate  UpperLimit=1  LowerLimit=-1
  Out1 : Outport
  wires:
  Ke1/1 -> e/1
  Kde1/1 -> Saturation1/1
  Derivative/1 -> Kde1/1
  In1/1 -> Derivative/1, Ke1/1
  e/1 -> PB/1, NB/1, ZE/1
  Saturation1/1 -> PB(1)/1, ZE(1)/1, NB(1)/1
  NB/1 -> NB-ZE(1)/1, NB-PB(1)/1, NB-NB(1)/1
  NB(1)/1 -> PB-NB(1)/2, NB-NB(1)/2, ZE-NB(1)/2
  ZE(1)/1 -> PB-ZE(1)/2, NB-ZE(1)/2, ZE-ZE(1)/2
  PB(1)/1 -> NB-PB(1)/2, ZE-PB(1)/2, PB-PB(1)/2
  ZE/1 -> ZE-NB(1)/1, ZE-ZE(1)/1, ZE-PB(1)/1
  PB/1 -> PB-NB(1)/1, PB-PB(1)/1, PB-ZE(1)/1
  NB-NB(1)/1 -> Add1/1, Gain1/1
  NB-ZE(1)/1 -> Add1/2, Gain/1
  NB-PB(1)/1 -> Add1/3, Gain2/1
  ZE-NB(1)/1 -> Add1/4, Gain3/1
  ZE-ZE(1)/1 -> Add1/5, Gain4/1
  ZE-PB(1)/1 -> Add1/6, Gain5/1
  PB-NB(1)/1 -> Add1/7, Gain6/1
  PB-ZE(1)/1 -> Add1/8, Gain7/1
  PB-PB(1)/1 -> Add1/9, Gain8/1
  Gain1/1 -> Add/1
  Gain/1 -> Add/2
  Gain2/1 -> Add/3
  Gain3/1 -> Add/4
  Gain4/1 -> Add/5
  Gain5/1 -> Add/6
  Gain6/1 -> Add/7
  Gain7/1 -> Add/8
  Gain8/1 -> Add/9
  Add/1 -> Product/1
  Add1/1 -> Product/2
  Integrator10/1 -> Ku1/1
  Product/1 -> Integrator10/1
  Ku1/1 -> Out1/1
